simulink subsystem "Battery"  (R2023b)
settings: Solver=VariableStepAuto  StartTime=0.0  StopTime=10.0  RelTol=1e-3
undefined symbols (not defined in the file): BatteryModelParams
settings Model: Creator=leona  LastModifiedBy=leona

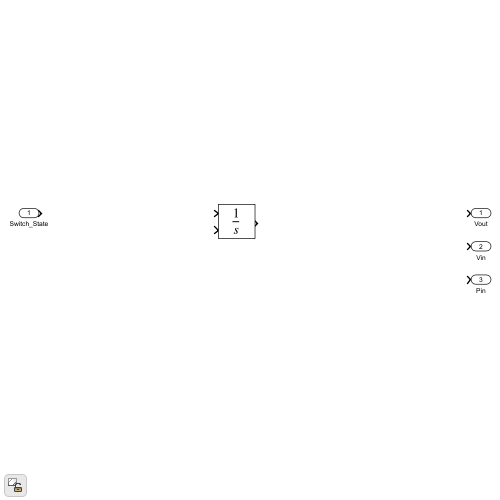
[thumbnail: Simulink's stored preview of the top-level diagram]
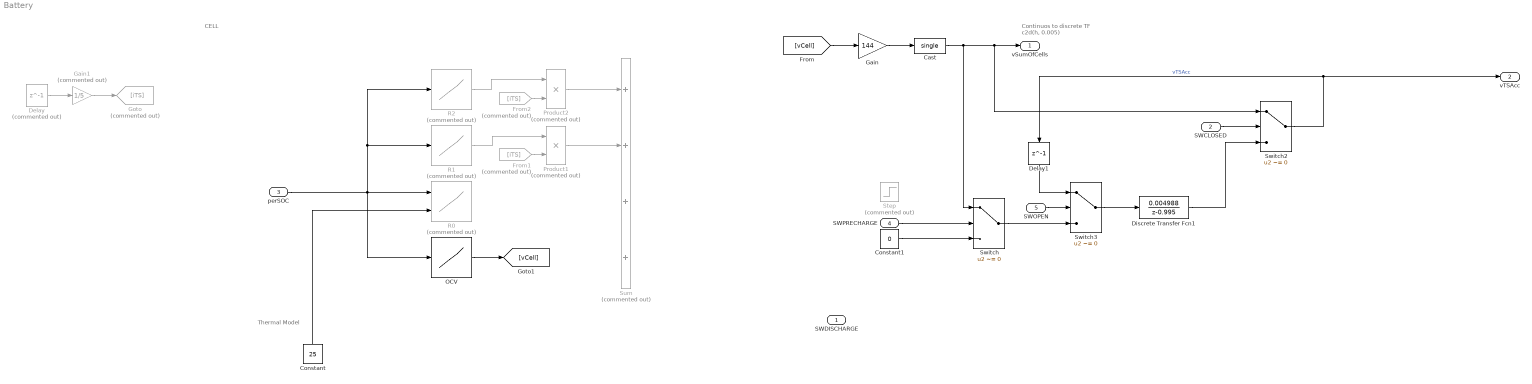
== system Battery ==
  note: CELL
  note: Thermal Model
  note: Continuos to discrete TF
      | c2d(h, 0.005)
  SWDISCHARGE : Inport
  SWCLOSED : Inport  Port=2
  perSOC : Inport  Port=3
  SWPRECHARGE : Inport  Port=4
  SWOPEN : Inport  Port=5
  Cast : DataTypeConversion  OutDataTypeStr=single  SaturateOnIntegerOverflow=off  RndMeth=Floor
  Constant : Constant  Value=25
  Constant1 : Constant  Value=0  OutDataTypeStr=single
  Delay : Delay  Commented=on  DelayLength=1
  Delay1 : Delay  DelayLength=1
  Discrete Transfer Fcn1 : DiscreteTransferFcn  Numerator=[0.004988]  Denominator=[1 -0.995]
  From1 : From  Commented=on  GotoTag=iTS
  From2 : From  Commented=on  GotoTag=iTS
  Gain : Gain  Gain=144  OutDataTypeStr=single
  Gain1 : Gain  Commented=on  Gain=1/5
  Goto : Goto  Commented=on  GotoTag=iTS
  OCV : Lookup_n-D  NumberOfTableDimensions=1  BreakpointsForDimension1=[1:100]  Table=BatteryModelParams.OCV_lut(:,1)  ExtrapMethod=Clip  InternalRulePriority=Speed  RndMeth=Simplest
  Product1 : Product  Commented=on
  Product2 : Product  Commented=on
  R0 : Lookup_n-D  Commented=on  BreakpointsForDimension1=[1:100]  BreakpointsForDimension2=[21:60]  Table=BatteryModelParams.R0_lut  InternalRulePriority=Speed  RndMeth=Simplest
      settings: InputPortMap=u0,u1
  R1 : Lookup_n-D  Commented=on  NumberOfTableDimensions=1  BreakpointsForDimension1=[1:100]  Table=BatteryModelParams.R1_lut(:,1)  InternalRulePriority=Speed  RndMeth=Simplest
  R2 : Lookup_n-D  Commented=on  NumberOfTableDimensions=1  BreakpointsForDimension1=[1:100]  Table=BatteryModelParams.C1_lut(:,1)  InternalRulePriority=Speed  RndMeth=Simplest
  Step : Step  Commented=on  Time=5  Before=1  After=0
  Sum : Sum  Commented=on  Inputs=++++
  Switch : Switch  Criteria=u2 ~= 0  SaturateOnIntegerOverflow=off  InputSameDT=off
  Switch2 : Switch  Criteria=u2 ~= 0  SaturateOnIntegerOverflow=off  InputSameDT=off
  Switch3 : Switch  Criteria=u2 ~= 0  SaturateOnIntegerOverflow=off  InputSameDT=off
  vSumOfCells : Outport
  vTSAcc : Outport  Port=2
  wires:
  Constant/1 -> R0/2
  perSOC/1 -> R0/1, R2/1, R1/1, OCV/1
  From1/1 -> Product1/2
  From2/1 -> Product2/2
  R2/1 -> Product2/1
  R1/1 -> Product1/1
  Product2/1 -> Sum/1
  Product1/1 -> Sum/2
  OCV/1 -> [vCell]
  Gain1/1 -> Goto/1
  Delay/1 -> Gain1/1
  [vCell] -> Gain/1
  Gain/1 -> Cast/1
  Cast/1 -> vSumOfCells/1, Switch2/1, Switch/1
  SWCLOSED/1 -> Switch2/2
  Switch2/1 -> Delay1/1, vTSAcc/1  "vTSAcc"
  Discrete Transfer Fcn1/1 -> Switch2/3
  SWOPEN/1 -> Switch3/2
  Switch3/1 -> Discrete Transfer Fcn1/1
  Delay1/1 -> Switch3/1
  Switch/1 -> Switch3/3
  Constant1/1 -> Switch/3
  SWPRECHARGE/1 -> Switch/2
